simulink model "demoDINA_PCS"  (Simulink 8.0)
settings: Solver=FixedStepDiscrete  SolverMode=SingleTasking  StartTime=80.0  StopTime=80.05  FixedStep=0.005  RelTol=1e-3
InitFcn:
  | init_param_PCS;
undefined symbols (not defined in the file or in its folder): PCSmatlab
libraries: simulink x1
settings Model: Creator=invite  LastModifiedBy=huynhp  ExtModeAutoUpdateStatusClock=off  TunableVars=K,num  TunableVarsStorageClass=Auto,Auto  TunableVarsTypeQualifier=,  BufferReuse=off
settings DataIOCC: SignalLoggingSaveFormat=ModelDataLogs
settings OptimizationCC: BlockReduction=off  BooleanDataType=off  ConditionallyExecuteInputs=off  OptimizeBlockIOStorage=off  BufferReuse=off  ExpressionFolding=off  LocalBlockOutputs=off  InitFltsAndDblsToZero=on  AccelVerboseBuild=on
settings DebuggingCC: FcnCallInpInsideContextMsg=UseLocalSettings  SFcnCompatibilityMsg=warning  StrictBusMsg=Warning
settings SFSimCC: SimBuildMode=sf_make
settings GRTTargetCC: CombineOutputUpdateFcns=off  GRTInterface=on

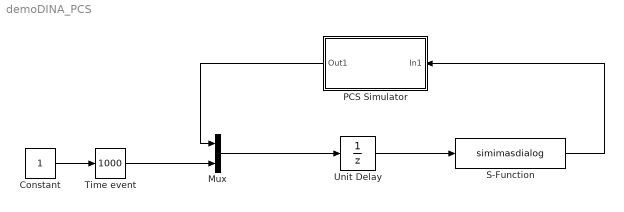
== system demoDINA_PCS ==
  Constant : Constant  SampleTime=-1
  Mux : Mux  Inputs=2
  PCS Simulator : Subsystem
  S-Function : S-Function  FunctionName=simimasdialog  EnableBusSupport=off
  Time event : simulink/Math Operations/Slider Gain  low=0  gain=1000  high=1000
  Unit Delay : UnitDelay  SampleTime=-1
  wires:
  Constant/1 -> Time event/1
  Unit Delay/1 -> S-Function/1
  Time event/1 -> Mux/2
  Mux/1 -> Unit Delay/1
  S-Function/1 -> PCS Simulator/1(In1)
  PCS Simulator/1(Out1) -> Mux/1

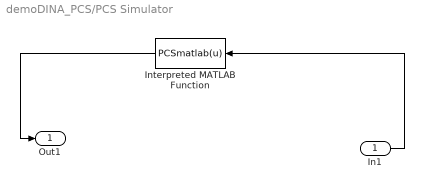
== system demoDINA_PCS/PCS Simulator ==
  In1 : Inport
  Interpreted MATLAB Function : MATLABFcn  MATLABFcn=PCSmatlab(u)  OutputDimensions=150
  Out1 : Outport
  wires:
  In1/1 -> Interpreted MATLAB Function/1
  Interpreted MATLAB Function/1 -> Out1/1
